simulink model "servo"  (R2017b)
settings: Solver=VariableStepAuto  StartTime=0.0  StopTime=10.0  RelTol=1e-3
settings Model: Creator=Bailey Brookes  LastModifiedBy=Bailey Brookes

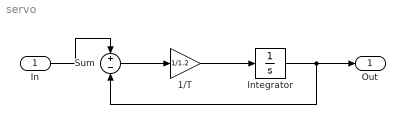
== system servo ==
  In : Inport
  1/T : Gain  Gain=1/1.2
  Integrator : Integrator
  Sum : Sum  Inputs=+-
  Out : Outport
  wires:
  In/1 -> Sum/1
  Sum/1 -> 1/T/1
  1/T/1 -> Integrator/1
  Integrator/1 -> Sum/2, Out/1
